simulink model "parte4_eje2_Thidraulica_mdl"  (R2017b)
settings: Solver=VariableStepAuto  StartTime=0.0  StopTime=100  RelTol=1e-3
values from neighbouring files (symbols this model uses):
  At = 1/(gFL-gNL)    (= 1.25)    [parte4_ej1_ThidraulicaNLdata.m]    (also in parte4_eje2_Thidraulica_const.m)
  CI = 10    [parte4_eje2_Thidraulica_const.m]
  gFL = 0.96    [parte4_ej1_ThidraulicaNLdata.m]    (also in parte4_eje2_Thidraulica_const.m)
  gNL = 0.16    [parte4_ej1_ThidraulicaNLdata.m]    (also in parte4_eje2_Thidraulica_const.m)
  Ho = 1    [parte4_ej1_ThidraulicaNLdata.m]    (also in parte4_eje2_Thidraulica_const.m)
  PR = 1    [parte4_eje2_Thidraulica_const.m]
  TW = 1    [parte4_ej1_ThidraulicaNLdata.m]    (also in parte4_eje2_Thidraulica_const.m)
  UNL = 0.068    [parte4_ej1_ThidraulicaNLdata.m]    (also in parte4_eje2_Thidraulica_const.m = 0.08)
  w = 1    [parte4_ej1_ThidraulicaNLdata.m]    (also in parte4_eje2_Thidraulica_const.m)
settings Model: Creator=cjuar  LastModifiedBy=Admon

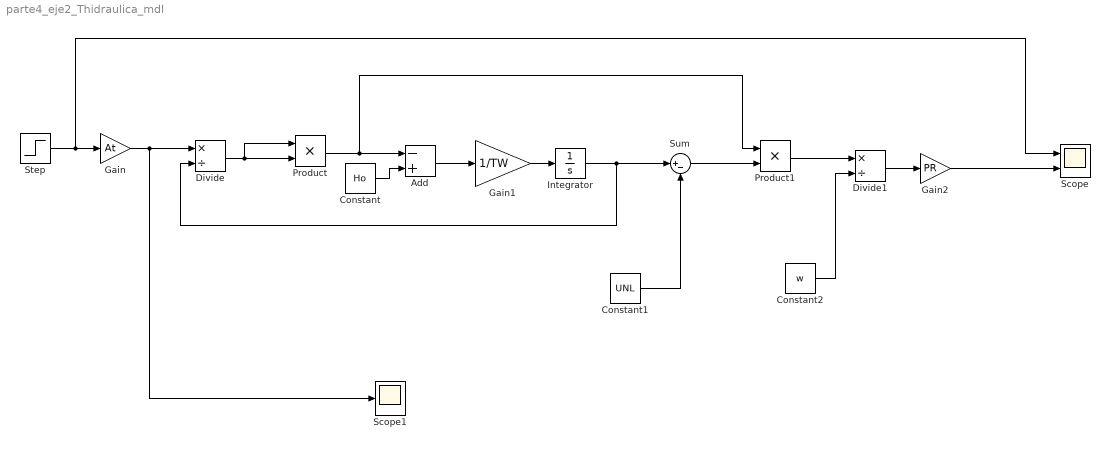
== system parte4_eje2_Thidraulica_mdl ==
  Add : Sum  Inputs=-+
  Constant : Constant  Value=Ho
  Constant1 : Constant  Value=UNL
  Constant2 : Constant  Value=w
  Divide : Product  Inputs=*/
  Divide1 : Product  Inputs=*/
  Gain : Gain  Gain=At
  Gain1 : Gain  Gain=1/TW
  Gain2 : Gain  Gain=PR
  Integrator : Integrator  InitialCondition=CI
  Product : Product
  Product1 : Product
  Scope : Scope  NumInputPorts=2
  Scope1 : Scope
  Step : Step  Time=5  Before=gNL  After=gFL  SampleTime=0
  Sum : Sum  Inputs=|+-
  wires:
  Gain/1 -> Scope1/1, Divide/1
  Divide/1 -> Product/1, Product/2
  Product/1 -> Product1/1, Add/1
  Constant/1 -> Add/2
  Add/1 -> Gain1/1
  Gain1/1 -> Integrator/1
  Integrator/1 -> Sum/1, Divide/2
  Constant1/1 -> Sum/2
  Sum/1 -> Product1/2
  Constant2/1 -> Divide1/2
  Divide1/1 -> Gain2/1
  Step/1 -> Scope/1, Gain/1
  Gain2/1 -> Scope/2
  Product1/1 -> Divide1/1
